simulink model "Local"  (R2024b)
settings: Solver=VariableStepAuto  StartTime=0.0  StopTime=10  RelTol=1e-3
undefined symbols (not defined in the file): A, A0_obv, Aa_obv, adj, agent_0, agent_1, agent_2, agent_3, agent_4, agent_5, agent_6, B, B0_obv, Ba_obv, c, C, C0_obv, Ca_obv, D, D0_obv, Da_obv, G, K, K0, leader_noise_variance
settings Model: Creator=39393  LastModifiedBy=Ivan

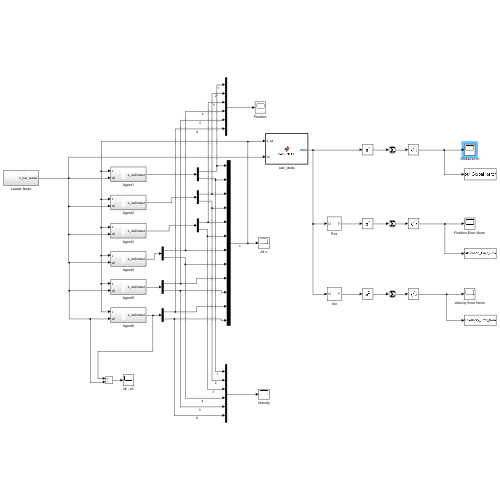
[thumbnail: Simulink's stored preview of the top-level diagram]
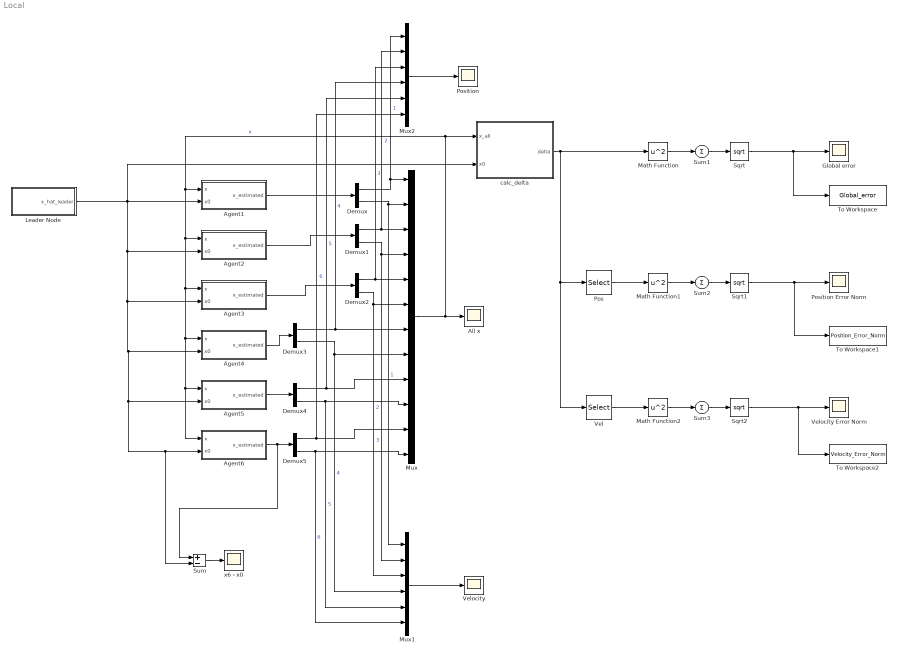
== system Local ==
  Agent1 : Subsystem
  Agent2 : Subsystem
  Agent3 : Subsystem
  Agent4 : Subsystem
  Agent5 : Subsystem
  Agent6 : Subsystem
  All x : Scope
  Demux{,1..5} (6 alike) : Demux  Outputs=2
  Global error : Scope
  Leader Node : Subsystem
  Math Function : Math  Operator=square
  Math Function1 : Math  Operator=square
  Math Function2 : Math  Operator=square
  Mux : Mux  Inputs=12
  Mux1 : Mux  Inputs=6
  Mux2 : Mux  Inputs=6
  Pos : Selector  NumberOfDimensions=2  InputPortWidth=3  IndexOptions=Index vector (dialog),Select all  Indices=[1],1  OutputSizes=1,1
  Position : Scope
  "Position Error Norm " : Scope
  Sqrt : Sqrt
  Sqrt1 : Sqrt
  Sqrt2 : Sqrt
  Sum : Sum  Inputs=+-
  Sum1 : Sum  Inputs=1
  Sum2 : Sum  Inputs=1
  Sum3 : Sum  Inputs=1
  To Workspace : ToWorkspace  VariableName=Global_error  SampleTime=-1
      settings: Save2DSignal=2-D array (concatenate along first dimension)
  To Workspace1 : ToWorkspace  VariableName=Position_Error_Norm  SampleTime=-1
      settings: Save2DSignal=2-D array (concatenate along first dimension)
  To Workspace2 : ToWorkspace  VariableName=Velocity_Error_Norm  SampleTime=-1
      settings: Save2DSignal=2-D array (concatenate along first dimension)
  Vel : Selector  NumberOfDimensions=2  InputPortWidth=3  IndexOptions=Index vector (dialog),Select all  Indices=[2],1  OutputSizes=1,1
  Velocity : Scope
  Velocity Error Norm : Scope
  calc_delta : MATLAB Function  TreatAsAtomicUnit=on
  x6 - x0 : Scope
  wires:
  Leader Node/1(x_hat_leader) -> calc_delta/2(x0), Agent5/2(x0), Agent6/2(x0), Sum/2, Agent4/2(x0), Agent3/2(x0), Agent2/2(x0), Agent1/2(x0)
  Agent1/1(x_estimated) -> Demux/1
  Mux/1 -> All x/1, calc_delta/1(x_all), Agent2/1(x), Agent3/1(x), Agent4/1(x), Agent5/1(x), Agent6/1(x), Agent1/1(x)  "x"
  Demux/1 -> Mux/1, Mux2/1  "1"
  Demux/2 -> Mux/2, Mux1/1  "1"
  Demux1/1 -> Mux2/2, Mux/3  "2"
  Demux1/2 -> Mux1/2, Mux/4  "2"
  Mux2/1 -> Position/1
  Mux1/1 -> Velocity/1
  Agent2/1(x_estimated) -> Demux1/1
  Agent3/1(x_estimated) -> Demux2/1
  Demux2/1 -> Mux/5, Mux2/3  "3"
  Demux2/2 -> Mux1/3, Mux/6  "3"
  Agent4/1(x_estimated) -> Demux3/1
  Demux3/1 -> Mux2/4, Mux/7  "4"
  Demux3/2 -> Mux1/4, Mux/8  "4"
  Agent5/1(x_estimated) -> Demux4/1
  Agent6/1(x_estimated) -> Sum/1, Demux5/1
  Demux4/1 -> Mux2/5, Mux/9  "5"
  Demux4/2 -> Mux1/5, Mux/10  "5"
  Demux5/1 -> Mux2/6, Mux/11  "6"
  Demux5/2 -> Mux1/6, Mux/12  "6"
  Sum/1 -> x6 - x0/1
  calc_delta/1(delta) -> Vel/1, Pos/1, Math Function/1
  Math Function/1 -> Sum1/1
  Sum1/1 -> Sqrt/1
  Pos/1 -> Math Function1/1
  Vel/1 -> Math Function2/1
  Math Function1/1 -> Sum2/1
  Math Function2/1 -> Sum3/1
  Sum2/1 -> Sqrt1/1
  Sum3/1 -> Sqrt2/1
  Sqrt1/1 -> To Workspace1/1, "Position Error Norm "/1
  Sqrt2/1 -> To Workspace2/1, Velocity Error Norm/1
  Sqrt/1 -> To Workspace/1, Global error/1

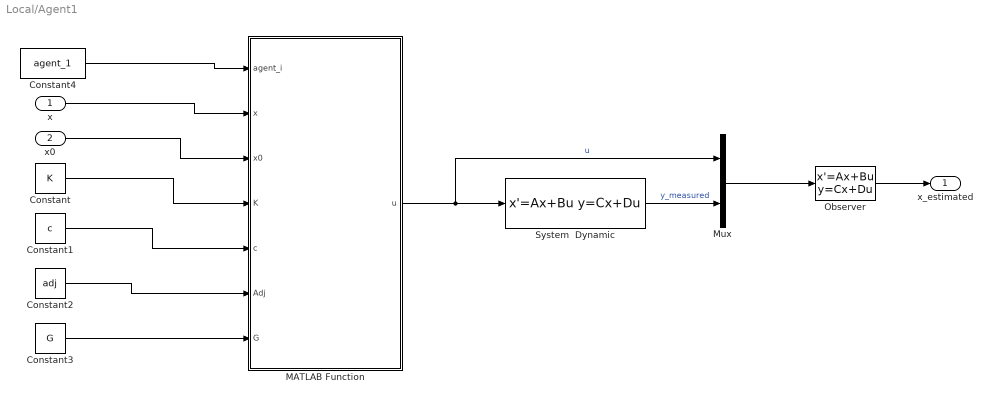
== system Local/Agent1 ==
  x : Inport
  x0 : Inport  Port=2
  Constant : Constant  Value=K  VectorParams1D=off
  Constant1 : Constant  Value=c
  Constant2 : Constant  Value=adj
  Constant3 : Constant  Value=G
  Constant4 : Constant  Value=agent_1  VectorParams1D=off
  MATLAB Function : MATLAB Function  TreatAsAtomicUnit=on
  Mux : Mux  Inputs=2
  Observer : StateSpace  A=Aa_obv  B=Ba_obv  C=Ca_obv  D=Da_obv  InitialCondition=0
  System  Dynamic : StateSpace  A=(A-B*K0)  B=B  C=C  D=0  InitialCondition=0
  x_estimated : Outport
  wires:
  x/1 -> MATLAB Function/2(x)
  Constant3/1 -> MATLAB Function/7(G)
  Constant1/1 -> MATLAB Function/5(c)
  Constant/1 -> MATLAB Function/4(K)
  Constant4/1 -> MATLAB Function/1(agent_i)
  Constant2/1 -> MATLAB Function/6(Adj)
  MATLAB Function/1(u) -> Mux/1, System  Dynamic/1  "u"
  System  Dynamic/1 -> Mux/2  "y_measured"
  Mux/1 -> Observer/1
  Observer/1 -> x_estimated/1
  x0/1 -> MATLAB Function/3(x0)

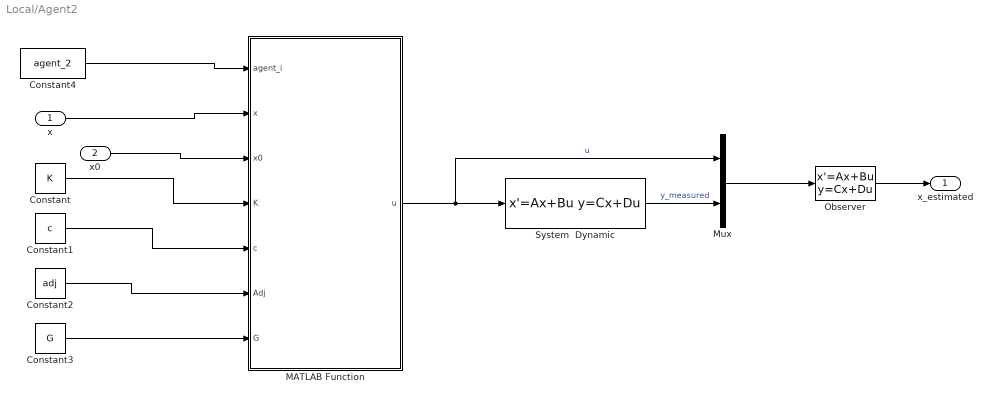
== system Local/Agent2 ==
  x : Inport
  x0 : Inport  Port=2
  Constant : Constant  Value=K  VectorParams1D=off
  Constant1 : Constant  Value=c
  Constant2 : Constant  Value=adj
  Constant3 : Constant  Value=G
  Constant4 : Constant  Value=agent_2  VectorParams1D=off
  MATLAB Function : MATLAB Function  TreatAsAtomicUnit=on
  Mux : Mux  Inputs=2
  Observer : StateSpace  A=Aa_obv  B=Ba_obv  C=Ca_obv  D=Da_obv  InitialCondition=0
  System  Dynamic : StateSpace  A=(A-B*K0)  B=B  C=C  D=0  InitialCondition=0
  x_estimated : Outport
  wires:
  x/1 -> MATLAB Function/2(x)
  Constant3/1 -> MATLAB Function/7(G)
  Constant1/1 -> MATLAB Function/5(c)
  Constant/1 -> MATLAB Function/4(K)
  Constant4/1 -> MATLAB Function/1(agent_i)
  Constant2/1 -> MATLAB Function/6(Adj)
  MATLAB Function/1(u) -> Mux/1, System  Dynamic/1  "u"
  System  Dynamic/1 -> Mux/2  "y_measured"
  Mux/1 -> Observer/1
  Observer/1 -> x_estimated/1
  x0/1 -> MATLAB Function/3(x0)

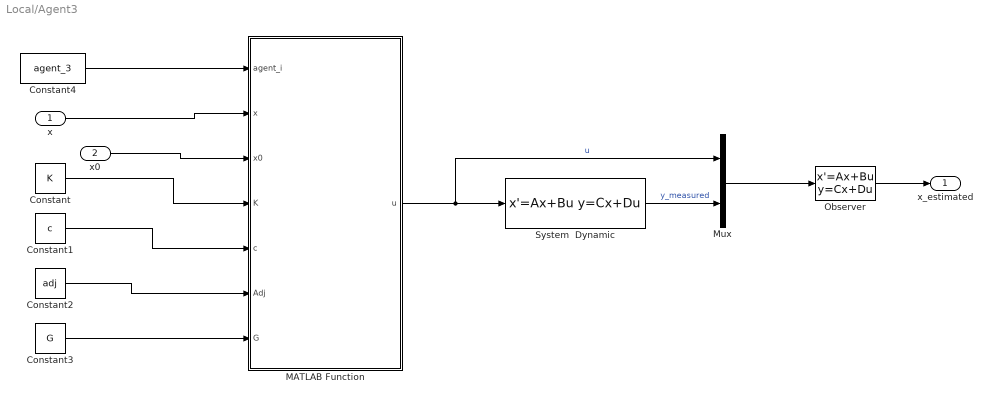
== system Local/Agent3 ==
  x : Inport
  x0 : Inport  Port=2
  Constant : Constant  Value=K  VectorParams1D=off
  Constant1 : Constant  Value=c
  Constant2 : Constant  Value=adj
  Constant3 : Constant  Value=G
  Constant4 : Constant  Value=agent_3  VectorParams1D=off
  MATLAB Function : MATLAB Function  TreatAsAtomicUnit=on
  Mux : Mux  Inputs=2
  Observer : StateSpace  A=Aa_obv  B=Ba_obv  C=Ca_obv  D=Da_obv  InitialCondition=0
  System  Dynamic : StateSpace  A=(A-B*K0)  B=B  C=C  D=0  InitialCondition=0
  x_estimated : Outport
  wires:
  x/1 -> MATLAB Function/2(x)
  Constant3/1 -> MATLAB Function/7(G)
  Constant1/1 -> MATLAB Function/5(c)
  Constant/1 -> MATLAB Function/4(K)
  Constant4/1 -> MATLAB Function/1(agent_i)
  Constant2/1 -> MATLAB Function/6(Adj)
  MATLAB Function/1(u) -> Mux/1, System  Dynamic/1  "u"
  System  Dynamic/1 -> Mux/2  "y_measured"
  Mux/1 -> Observer/1
  Observer/1 -> x_estimated/1
  x0/1 -> MATLAB Function/3(x0)

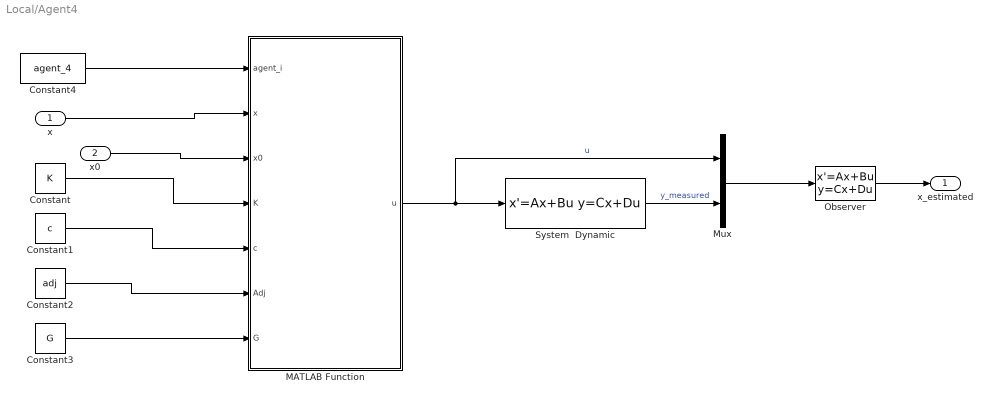
== system Local/Agent4 ==
  x : Inport
  x0 : Inport  Port=2
  Constant : Constant  Value=K  VectorParams1D=off
  Constant1 : Constant  Value=c
  Constant2 : Constant  Value=adj
  Constant3 : Constant  Value=G
  Constant4 : Constant  Value=agent_4  VectorParams1D=off
  MATLAB Function : MATLAB Function  TreatAsAtomicUnit=on
  Mux : Mux  Inputs=2
  Observer : StateSpace  A=Aa_obv  B=Ba_obv  C=Ca_obv  D=Da_obv  InitialCondition=0
  System  Dynamic : StateSpace  A=(A-B*K0)  B=B  C=C  D=0  InitialCondition=0
  x_estimated : Outport
  wires:
  x/1 -> MATLAB Function/2(x)
  Constant3/1 -> MATLAB Function/7(G)
  Constant1/1 -> MATLAB Function/5(c)
  Constant/1 -> MATLAB Function/4(K)
  Constant4/1 -> MATLAB Function/1(agent_i)
  Constant2/1 -> MATLAB Function/6(Adj)
  MATLAB Function/1(u) -> Mux/1, System  Dynamic/1  "u"
  System  Dynamic/1 -> Mux/2  "y_measured"
  Mux/1 -> Observer/1
  Observer/1 -> x_estimated/1
  x0/1 -> MATLAB Function/3(x0)

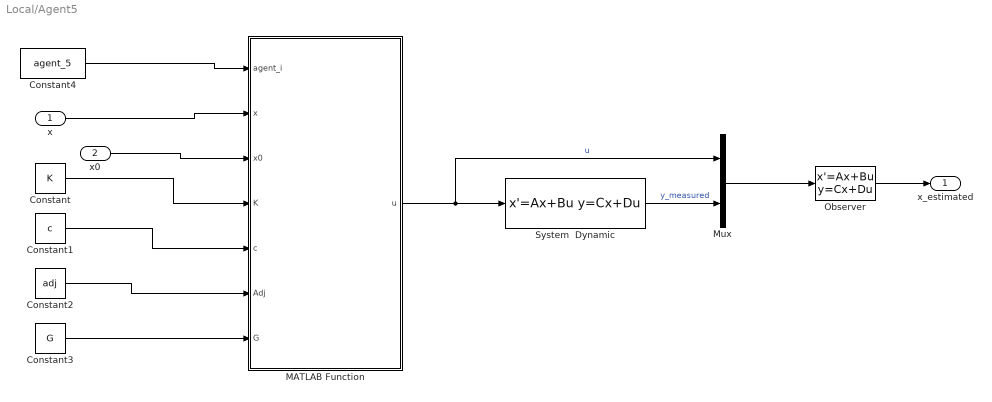
== system Local/Agent5 ==
  x : Inport
  x0 : Inport  Port=2
  Constant : Constant  Value=K  VectorParams1D=off
  Constant1 : Constant  Value=c
  Constant2 : Constant  Value=adj
  Constant3 : Constant  Value=G
  Constant4 : Constant  Value=agent_5  VectorParams1D=off
  MATLAB Function : MATLAB Function  TreatAsAtomicUnit=on
  Mux : Mux  Inputs=2
  Observer : StateSpace  A=Aa_obv  B=Ba_obv  C=Ca_obv  D=Da_obv  InitialCondition=0
  System  Dynamic : StateSpace  A=(A-B*K0)  B=B  C=C  D=0  InitialCondition=0
  x_estimated : Outport
  wires:
  x/1 -> MATLAB Function/2(x)
  Constant3/1 -> MATLAB Function/7(G)
  Constant1/1 -> MATLAB Function/5(c)
  Constant/1 -> MATLAB Function/4(K)
  Constant4/1 -> MATLAB Function/1(agent_i)
  Constant2/1 -> MATLAB Function/6(Adj)
  MATLAB Function/1(u) -> Mux/1, System  Dynamic/1  "u"
  System  Dynamic/1 -> Mux/2  "y_measured"
  Mux/1 -> Observer/1
  Observer/1 -> x_estimated/1
  x0/1 -> MATLAB Function/3(x0)

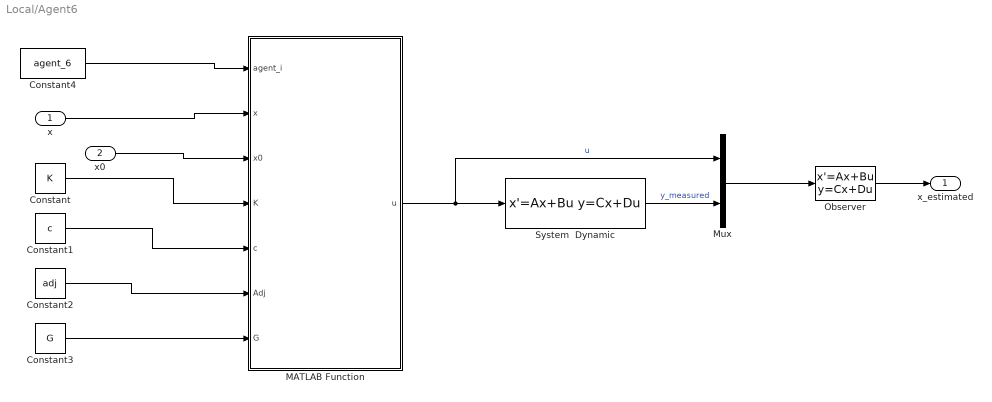
== system Local/Agent6 ==
  x : Inport
  x0 : Inport  Port=2
  Constant : Constant  Value=K  VectorParams1D=off
  Constant1 : Constant  Value=c
  Constant2 : Constant  Value=adj
  Constant3 : Constant  Value=G
  Constant4 : Constant  Value=agent_6  VectorParams1D=off
  MATLAB Function : MATLAB Function  TreatAsAtomicUnit=on
  Mux : Mux  Inputs=2
  Observer : StateSpace  A=Aa_obv  B=Ba_obv  C=Ca_obv  D=Da_obv  InitialCondition=0
  System  Dynamic : StateSpace  A=(A-B*K0)  B=B  C=C  D=0  InitialCondition=0
  x_estimated : Outport
  wires:
  x/1 -> MATLAB Function/2(x)
  Constant3/1 -> MATLAB Function/7(G)
  Constant1/1 -> MATLAB Function/5(c)
  Constant/1 -> MATLAB Function/4(K)
  Constant4/1 -> MATLAB Function/1(agent_i)
  Constant2/1 -> MATLAB Function/6(Adj)
  MATLAB Function/1(u) -> Mux/1, System  Dynamic/1  "u"
  System  Dynamic/1 -> Mux/2  "y_measured"
  Mux/1 -> Observer/1
  Observer/1 -> x_estimated/1
  x0/1 -> MATLAB Function/3(x0)

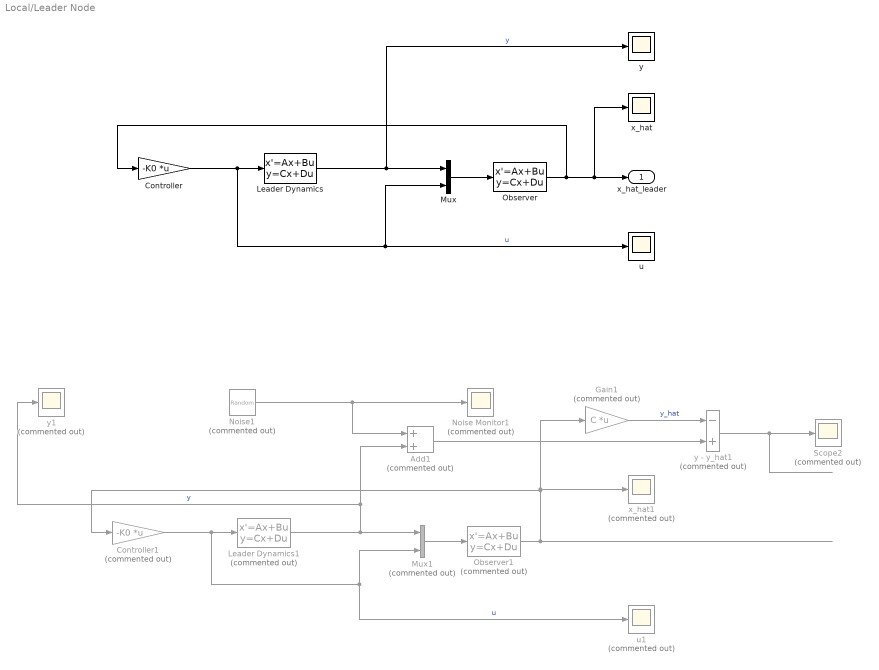
== system Local/Leader Node ==
  Add1 : Sum  Commented=on
  Controller : Gain  Gain=-K0  Multiplication=Matrix(K*u)
  Controller1 : Gain  Commented=on  Gain=-K0  Multiplication=Matrix(K*u)
  Gain1 : Gain  Commented=on  Gain=C  Multiplication=Matrix(K*u)
  Leader Dynamics : StateSpace  A=A  B=B  C=C  D=D  InitialCondition=[0 100]'
  Leader Dynamics1 : StateSpace  Commented=on  A=A  B=B  C=C  D=D  InitialCondition=[0 10]'
  Mux : Mux  Inputs=2
  Mux1 : Mux  Commented=on  Inputs=2
  Noise Monitor1 : Scope  Commented=on
  Noise1 : RandomNumber  Commented=on  Variance=leader_noise_variance  Seed=agent_0  SampleTime=0.01
  Observer : StateSpace  A=A0_obv  B=B0_obv  C=C0_obv  D=D0_obv  InitialCondition=0
  Observer1 : StateSpace  Commented=on  A=A0_obv  B=B0_obv  C=C0_obv  D=D0_obv  InitialCondition=0
  Scope2 : Scope  Commented=on
  u : Scope
  u1 : Scope  Commented=on
  x_hat : Scope
  x_hat1 : Scope  Commented=on
  y : Scope
  y - y_hat1 : Sum  Commented=on  Inputs=-+
  y1 : Scope  Commented=on
  x_hat_leader : Outport
  wires:
  Controller/1 -> Leader Dynamics/1, u/1, Mux/2  "u"
  Leader Dynamics/1 -> y/1, Mux/1  "y"
  Mux/1 -> Observer/1
  Observer/1 -> Controller/1, x_hat/1, x_hat_leader/1
  y - y_hat1/1 -> Scope2/1
  Controller1/1 -> Leader Dynamics1/1, u1/1, Mux1/2  "u"
  Observer1/1 -> x_hat1/1, Gain1/1, Controller1/1
  Add1/1 -> y - y_hat1/2
  Noise1/1 -> Add1/1, Noise Monitor1/1
  Mux1/1 -> Observer1/1
  Gain1/1 -> y - y_hat1/1  "y_hat"
  Leader Dynamics1/1 -> Add1/2, y1/1, Mux1/1  "y"

== matlab function Local/Agent2/MATLAB Function ==
  data: agent_i input; u output; x input; x0 input; K input; c input; Adj input; G input
function u = controller_agent(agent_i, x, x0, K, c, Adj, G)

% N = number of agents
N = length(Adj);  

% Number of entries of x
order = 2;

% Get the i-th 2x1 vector from the 12x1 size array (12 = N * 2, without leader)
get_x = @(idx) x(idx*order - (order-1) : idx*order);

% Error towards leader (reference)
a = G(agent_i)*(x0 - get_x(agent_i));

% Consensus error among agents
epsilon_i = zeros(order, 1);
for j = 1:N
    epsilon_i = epsilon_i + Adj(agent_i, j) * (get_x(j) - get_x(agent_i));
end

% Total error
epsilon_i = epsilon_i + a;

% Control law
u = c*K*epsilon_i;

== matlab function Local/Agent1/MATLAB Function ==
  data: agent_i input; u output; x input; x0 input; K input; c input; Adj input; G input
function u = controller_agent(agent_i, x, x0, K, c, Adj, G)

% N = number of agents
N = length(Adj);  

% Number of entries of x
order = 2;

% Get the i-th 2x1 vector from the 12x1 size array (12 = N * 2, without leader)
get_x = @(idx) x(idx*order - (order-1) : idx*order);

% Error towards leader (reference)
a = G(agent_i)*(x0 - get_x(agent_i));

% Consensus error among agents
epsilon_i = zeros(order, 1);
for j = 1:N
    epsilon_i = epsilon_i + Adj(agent_i, j) * (get_x(j) - get_x(agent_i));
end

% Total error
epsilon_i = epsilon_i + a;

% Control law
u = c*K*epsilon_i;

== matlab function Local/Agent3/MATLAB Function ==
  data: agent_i input; u output; x input; x0 input; K input; c input; Adj input; G input
function u = controller_agent(agent_i, x, x0, K, c, Adj, G)

% N = number of agents
N = length(Adj);  

% Number of entries of x
order = 2;

% Get the i-th 2x1 vector from the 12x1 size array (12 = N * 2, without leader)
get_x = @(idx) x(idx*order - (order-1) : idx*order);

% Error towards leader (reference)
a = G(agent_i)*(x0 - get_x(agent_i));

% Consensus error among agents
epsilon_i = zeros(order, 1);
for j = 1:N
    epsilon_i = epsilon_i + Adj(agent_i, j) * (get_x(j) - get_x(agent_i));
end

% Total error
epsilon_i = epsilon_i + a;

% Control law
u = c*K*epsilon_i;

== matlab function Local/Agent4/MATLAB Function ==
  data: agent_i input; u output; x input; x0 input; K input; c input; Adj input; G input
function u = controller_agent(agent_i, x, x0, K, c, Adj, G)

% N = number of agents
N = length(Adj);  

% Number of entries of x
order = 2;

% Get the i-th 2x1 vector from the 12x1 size array (12 = N * 2, without leader)
get_x = @(idx) x(idx*order - (order-1) : idx*order);

% Error towards leader (reference)
a = G(agent_i)*(x0 - get_x(agent_i));

% Consensus error among agents
epsilon_i = zeros(order, 1);
for j = 1:N
    epsilon_i = epsilon_i + Adj(agent_i, j) * (get_x(j) - get_x(agent_i));
end

% Total error
epsilon_i = epsilon_i + a;

% Control law
u = c*K*epsilon_i;

== matlab function Local/Agent5/MATLAB Function ==
  data: agent_i input; u output; x input; x0 input; K input; c input; Adj input; G input
function u = controller_agent(agent_i, x, x0, K, c, Adj, G)

% N = number of agents
N = length(Adj);  

% Number of entries of x
order = 2;

% Get the i-th 2x1 vector from the 12x1 size array (12 = N * 2, without leader)
get_x = @(idx) x(idx*order - (order-1) : idx*order);

% Error towards leader (reference)
a = G(agent_i)*(x0 - get_x(agent_i));

% Consensus error among agents
epsilon_i = zeros(order, 1);
for j = 1:N
    epsilon_i = epsilon_i + Adj(agent_i, j) * (get_x(j) - get_x(agent_i));
end

% Total error
epsilon_i = epsilon_i + a;

% Control law
u = c*K*epsilon_i;

== matlab function Local/Agent6/MATLAB Function ==
  data: agent_i input; u output; x input; x0 input; K input; c input; Adj input; G input
function u = controller_agent(agent_i, x, x0, K, c, Adj, G)

% N = number of agents
N = length(Adj);  

% Number of entries of x
order = 2;

% Get the i-th 2x1 vector from the 12x1 size array (12 = N * 2, without leader)
get_x = @(idx) x(idx*order - (order-1) : idx*order);

% Error towards leader (reference)
a = G(agent_i)*(x0 - get_x(agent_i));

% Consensus error among agents
epsilon_i = zeros(order, 1);
for j = 1:N
    epsilon_i = epsilon_i + Adj(agent_i, j) * (get_x(j) - get_x(agent_i));
end

% Total error
epsilon_i = epsilon_i + a;

% Control law
u = c*K*epsilon_i;

== matlab function Local/calc_delta ==
  data: x_all input; delta output; x0 input
function delta = calc_delta(x_all, x0)
% x_all: vettore [12x1] (2 stati per ciascuno dei 6 follower)
% x0: vettore [2x1] (leader)

N = length(x_all)/2; % numero di follower
delta = zeros(2, N); % matrice [2x6]

for i = 1:N
    xi = x_all(2*i-1:2*i); % prendi x_i
    delta(:, i) = xi - x0; % errore rispetto al leader
end

%Uscita del blocco delta:
%È una matrice 2×6 (righe = [posizione; velocità], colonne = agenti)
